simulink model "test1"  (R2022a)
settings: Solver=VariableStepAuto  StartTime=0.0  StopTime=25  RelTol=1e-3
libraries: spsDiodeLib x3, spsPVArrayLib x3, spsControlledVoltageSourceLib x1, spsCurrentMeasurementLib x1, simulink x1, spsVoltageMeasurementLib x1, spspowerguiLib x1
settings Model: Creator=Dell  LastModifiedBy=Dell

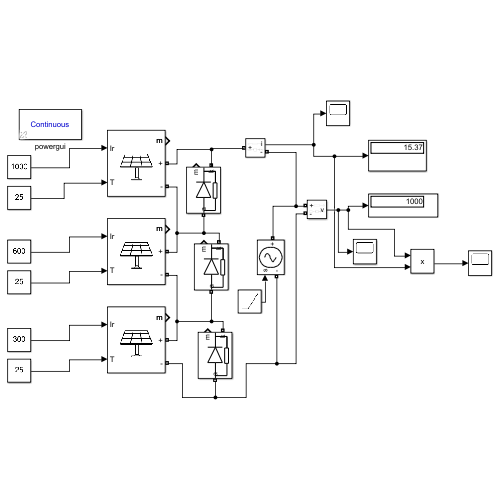
[thumbnail: Simulink's stored preview of the top-level diagram]
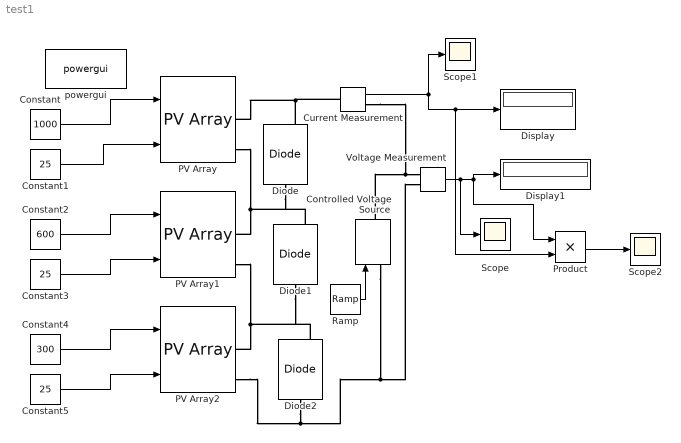
== system test1 ==
  Constant : Constant  Value=1000
  Constant1 : Constant  Value=25
  Constant2 : Constant  Value=600
  Constant3 : Constant  Value=25
  Constant4 : Constant  Value=300
  Constant5 : Constant  Value=25
  Controlled Voltage Source : spsControlledVoltageSourceLib/Controlled Voltage Source  Initialize=on  Source_Type=AC  Amplitude=0  Phase=0  Frequency=0  Measurements=None
  Current Measurement : spsCurrentMeasurementLib/Current Measurement  PhasorSimulation=off  OutputType=Complex  PSBequivalent=0
  Diode : spsDiodeLib/Diode  Ron=0.001  Lon=0  Vf=0.8  IC=0  UseSnubber=0  Rs=500  Cs=250e-9  Measurements=on
  Diode1 : spsDiodeLib/Diode  Ron=0.001  Lon=0  Vf=0.8  IC=0  UseSnubber=0  Rs=500  Cs=250e-9  Measurements=on
  Diode2 : spsDiodeLib/Diode  Ron=0.001  Lon=0  Vf=0.8  IC=0  UseSnubber=0  Rs=500  Cs=250e-9  Measurements=on
  Display : Display
  Display1 : Display
  PV Array : spsPVArrayLib/PV Array  Npar=10  Nser=10  PlotType=array @ 1000 W/m2 & specified temperatures  S_vec="[ 1000  500  100 ]"  Temp_C_vec="[ 45 25  ]"  ModuleName=Aavid Solar ASMS-165P  PlotWhenSelected=off  Pm=164.85  Ncell=72  Voc=43.5  Isc=5.25  Vm=35  Im=4.71  beta_Voc_pc=-0.393  alpha_Isc_pc=0.03  beta_Voc=-0.17095  alpha_Isc=0.001575  IL=5.2764  I0=4.9875e-10  nI=1.0218  Rsh=125.0069  Rs=0.62818  RobustModel=off  RobustCellTemperature=313.3991  BAL=on  Tc=1e-6  Tfilter=5e-5
  PV Array1 : spsPVArrayLib/PV Array  Npar=10  Nser=10  PlotType=array @ 1000 W/m2 & specified temperatures  S_vec="[ 1000  500  100 ]"  Temp_C_vec="[ 45 25  ]"  ModuleName=Aavid Solar ASMS-165P  PlotWhenSelected=off  Pm=164.85  Ncell=72  Voc=43.5  Isc=5.25  Vm=35  Im=4.71  beta_Voc_pc=-0.393  alpha_Isc_pc=0.03  beta_Voc=-0.17095  alpha_Isc=0.001575  IL=5.2764  I0=4.9875e-10  nI=1.0218  Rsh=125.0069  Rs=0.62818  RobustModel=off  RobustCellTemperature=313.3991  BAL=on  Tc=1e-6  Tfilter=5e-5
  PV Array2 : spsPVArrayLib/PV Array  Npar=10  Nser=10  PlotType=array @ 1000 W/m2 & specified temperatures  S_vec="[ 1000  500  100 ]"  Temp_C_vec="[ 45 25  ]"  ModuleName=Aavid Solar ASMS-165P  PlotWhenSelected=off  Pm=164.85  Ncell=72  Voc=43.5  Isc=5.25  Vm=35  Im=4.71  beta_Voc_pc=-0.393  alpha_Isc_pc=0.03  beta_Voc=-0.17095  alpha_Isc=0.001575  IL=5.2764  I0=4.9875e-10  nI=1.0218  Rsh=125.0069  Rs=0.62818  RobustModel=off  RobustCellTemperature=313.3991  BAL=on  Tc=1e-6  Tfilter=5e-5
  Product : Product
  Ramp : simulink/Sources/Ramp  slope=40  start=0  InitialOutput=0
  Scope : Scope
  Scope1 : Scope
  Scope2 : Scope
  Voltage Measurement : spsVoltageMeasurementLib/Voltage Measurement  PhasorSimulation=off  OutputType=Complex  PSBequivalent=0
  powergui : spspowerguiLib/powergui  Priority=1  SimulationMode=Continuous  SampleTime=50e-6  frequency=60  Iterations=50  frequencyindice=0  Pbase=100e6  ErrMax=1e-4  UnitsV=kV  UnitsW=MW  buscounter=0  FunctionMessages=off  echomessages=off  EnableUseOfTLC=off  CurrentSourceSwitches=off  DisableSnubberDevices=off  DisableRonSwitches=off  DisableVfSwitches=off  DisplayEquations=off  AutomaticDiscreteSolvers=off  SolverType=Tustin/Backward Euler (TBE)  Interpol=off  ExternalGateDelay=off  methode=off  Ts=100  x0status=blocks  SPID=on  SwTol=0  HookPort=off  NonlinearTolerance=1e-4  nMaxIteration=100  ContinueOnMaxIteration=off  RestoreLinks=warning  ResistiveCurrentMeasurement=off  Frange=[0:2:500]  Ylog=off  Xlog=on  ShowGrid=off  save=off  variable=ZData  structure=0  ZoomFFT=off  StartTime=0.0  cycles=1  DisplayStyle=1  fundamental=60  FreqAxis=off  MaxFrequency=1000  frequencyindicesteady=1  RmsSteady=1  display=off
  wires:
  Constant/1 -> PV Array/1
  Constant1/1 -> PV Array/2
  Current Measurement/1 -> Scope1/1, Product/2, Display/1
  Voltage Measurement/1 -> Scope/1, Product/1, Display1/1
  Constant2/1 -> PV Array1/1
  Constant3/1 -> PV Array1/2
  Constant4/1 -> PV Array2/1
  Constant5/1 -> PV Array2/2
  Ramp/1 -> Controlled Voltage Source/1
  Product/1 -> Scope2/1
  connections:
  Current Measurement/RConn1 -- Controlled Voltage Source/RConn1 -- Voltage Measurement/LConn1
  PV Array2/RConn2 -- Diode2/LConn1 -- Controlled Voltage Source/LConn1 -- Voltage Measurement/LConn2
  Diode/RConn1 -- Current Measurement/LConn1 -- PV Array/RConn1
  PV Array/RConn2 -- Diode1/RConn1 -- Diode/LConn1 -- PV Array1/RConn1
  PV Array1/RConn2 -- Diode2/RConn1 -- Diode1/LConn1 -- PV Array2/RConn1
